simulink model "GalvoModel_v3_siso_cl1"  (R2013a)
settings: Solver=ode45  StartTime=0.0  StopTime=1.5  RelTol=1e-3
undefined symbols (not defined in the file or in its folder): BEM, CL, CR, FR, H, KTR, RIN, TRC
libraries: simulink x1, cstblocks x1
settings Model: Creator=mainster  LastModifiedBy=mainster
settings DebuggingCC: SolverPrmCheckMsg=none

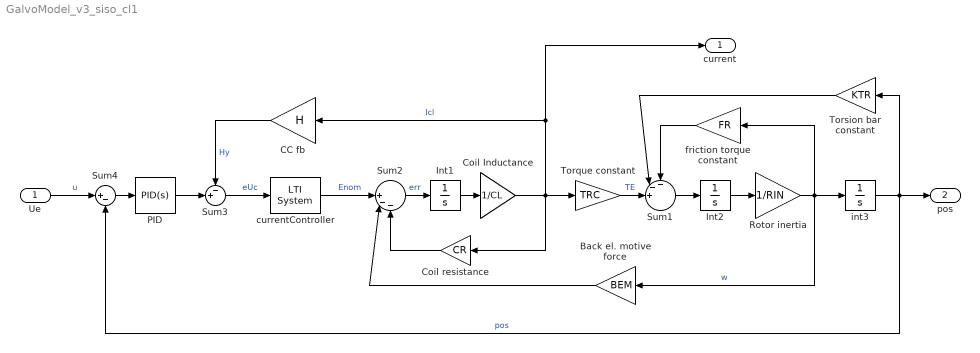
== system GalvoModel_v3_siso_cl1 ==
  Ue : Inport
  Back el. motive force : Gain  Gain=BEM
  CC fb : Gain  StartFcn=|  Gain=H
      | %H=100;                       
      | sprintf('StartFcn: H is %i',H)
      settings: AttributesFormatString=H=eval(%<Gain>)
  Coil Inductance : Gain  Gain=1/CL
  Coil resistance : Gain  Gain=CR
  Int1 : Integrator
  Int2 : Integrator
  PID : simulink/Continuous/PID Controller  Controller=PID  TimeDomain=Continuous-time  SampleTime=1  IntegratorMethod=Forward Euler  FilterMethod=Forward Euler  Form=Parallel  P=0.8254  I=0.7525  D=0.156  N=100  InitialConditionSource=internal  InitialConditionForIntegrator=0  InitialConditionForFilter=0  ExternalReset=none  LimitOutput=off  UpperSaturationLimit=inf  LowerSaturationLimit=-inf  LinearizeAsGain=on  AntiWindupMode=none  Kb=1  TrackingMode=off  Kt=1  PParamMin=[]  PParamMax=[]  IParamMin=[]  IParamMax=[]  DParamMin=[]  DParamMax=[]  NParamMin=[]  NParamMax=[]  KbParamMin=[]  KbParamMax=[]  KtParamMin=[]  KtParamMax=[]  POutMin=[]  POutMax=[]  IOutMin=[]  IOutMax=[]  DOutMin=[]  DOutMax=[]  NOutMin=[]  NOutMax=[]  KbOutMin=[]  KbOutMax=[]  KtOutMin=[]  KtOutMax=[]  IntegratorOutMin=[]  IntegratorOutMax=[]  FilterOutMin=[]  FilterOutMax=[]  SumOutMin=[]  SumOutMax=[]  SumI1OutMin=[]  SumI1OutMax=[]  SumI2OutMin=[]  SumI2OutMax=[]  SumI3OutMin=[]  SumI3OutMax=[]  SumDOutMin=[]  SumDOutMax=[]  SaturationOutMin=[]  SaturationOutMax=[]  IntegratorContinuousStateAttributes=''  IntegratorStateMustResolveToSignalObject=off  IntegratorRTWStateStorageClass=Auto  FilterContinuousStateAttributes=''  FilterStateMustResolveToSignalObject=off  FilterRTWStateStorageClass=Auto
  Rotor inertia : Gain  Gain=1/RIN
  Sum1 : Sum  Inputs=--+||
  Sum2 : Sum  Inputs=||+--
  Sum3 : Sum  Inputs=-+|
  Sum4 : Sum  Inputs=|+-
      settings: AttributesFormatString=%<Name>
  Torque constant : Gain  Gain=TRC
  Torsion bar constant : Gain  Gain=KTR
  currentController : cstblocks/LTI System  sys=zpk([-4336820.35478421;3315329.6730071],[-5399.66661710478+343615.713140898i;-5399.66661710478-343615.713140898i],-5.71084774711266,0)  IC=[]
  friction torque constant : Gain  Gain=FR
  int3 : Integrator
  current : Outport
  pos : Outport  Port=2
  wires:
  Sum2/1 -> Int1/1  "err"
  Rotor inertia/1 -> Back el. motive force/1, int3/1, friction torque constant/1  "w"
  int3/1 -> pos/1, Sum4/2, Torsion bar constant/1  "pos"
  Int1/1 -> Coil Inductance/1
  Coil resistance/1 -> Sum2/3
  Int2/1 -> Rotor inertia/1
  friction torque constant/1 -> Sum1/1
  Torsion bar constant/1 -> Sum1/2
  Torque constant/1 -> Sum1/3  "TE"
  Sum1/1 -> Int2/1
  Sum3/1 -> currentController/1  "eUc"
  currentController/1 -> Sum2/1  "Enom"
  Back el. motive force/1 -> Sum2/2
  Coil Inductance/1 -> current/1, CC fb/1, Coil resistance/1, Torque constant/1  "Icl"
  CC fb/1 -> Sum3/1  "Hy"
  PID/1 -> Sum3/2
  Sum4/1 -> PID/1
  Ue/1 -> Sum4/1  "u"
